simulink model "finalcode"  (R2020a)
settings: Solver=FixedStepDiscrete  StartTime=0.0  StopTime=1  FixedStep=0.0005  RelTol=1e-3  EnableMultiTasking=on
undefined symbols (not defined in the file): acc_calmax1, acc_calmax2, acc_calmin1, acc_calmin2, akemancanshu, angle_middle, bre, bre_calmax, bre_calmin, chasuniujvvvv_hou, chasuniujvvvv_qian, chasuuuu, ecucoder_acal, I_AN01_5K1, I_AN03_5V, I_AN04_5V, kd, kddd, ki, kiii, kp, kppp, leftmax, O_SW06_HS1A, P11111, P22222, PIDmodel, PPPP, rightmax, slip, slip_big, slip_little, slipmodel, T_add, T_del, tiaoshi, TTTTTyouren, vvvv, zhiling
libraries: ec5744lib x305, canmsglib x97, simulink x23
(part 5 of 11)

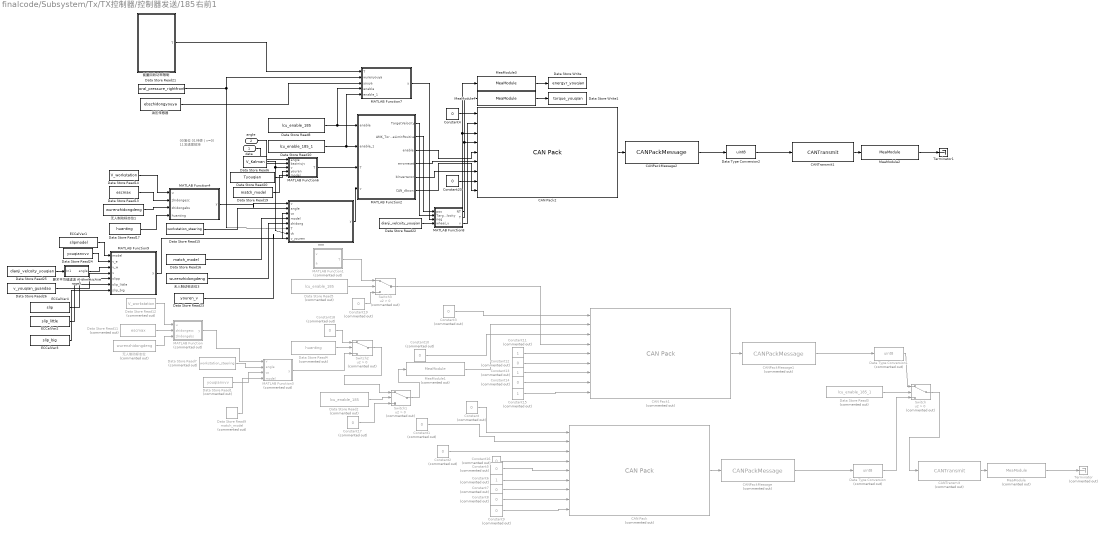
== system finalcode/Subsystem/Tx/TX控制器/控制器发送/185右前1 ==
  note: 00复位
      | 01待使（v=0)
      | 11发速度扭矩
  data : Inport
  angle : Inport  Port=2
  CAN Pack : canmsglib/CAN Pack  Commented=on  CANdbFile=D:\desktop\CANdbc\enable - youqian.dbc  MsgList=(none)  MsgName=first_enable  MsgIDType=Standard (11-bit identifier)  MsgIdentifier=389  MsgLength=8  Remote=off  ApplyMinMax=off  BusOutput=off  SignalInfo={'AMK_Reserve','12','4','LE','signed','Standard','0','1','0','0','15';'AMK_TargetVelocity','16','16','LE','signed','Standard','0','1','0','0','65535';'AMK_TorqueLimitNegativ','48','16','LE','signed','Standard','0','1','0','0','65535';'AMK_TorqueLimitPositiv','32','16','LE','signed','Standard','0','1','0','0','65535';'AMK_bEnable','10','1','LE','unsigned','Standard','0','1','0','0','1';'AMK_bErrorReset','11','1','LE','unsigned','Standard','0','1','0','0','1';'AMK_bInverterOn','8','1','LE','unsigned','Standard','0','1','0','0','1';'AMK_bReserve','0','8','LE','unsigned','Standard','0','1','0','0','255';'CAN_bdcon','9','1','LE','unsigned','Standard','0','1','0','0','1'}
      settings: SourceProductBaseCode=ME,XP,VN  DataFormat=CANdb specified signals
  CAN Pack1 : canmsglib/CAN Pack  Commented=on  CANdbFile=D:\desktop\CANdbc\enable - youqian.dbc  MsgList=(none)  MsgName=first_enable  MsgIDType=Standard (11-bit identifier)  MsgIdentifier=389  MsgLength=8  Remote=off  ApplyMinMax=off  BusOutput=off  SignalInfo={'AMK_Reserve','12','4','LE','signed','Standard','0','1','0','0','15';'AMK_TargetVelocity','16','16','LE','signed','Standard','0','1','0','0','65535';'AMK_TorqueLimitNegativ','48','16','LE','signed','Standard','0','1','0','0','65535';'AMK_TorqueLimitPositiv','32','16','LE','signed','Standard','0','1','0','0','65535';'AMK_bEnable','10','1','LE','unsigned','Standard','0','1','0','0','1';'AMK_bErrorReset','11','1','LE','unsigned','Standard','0','1','0','0','1';'AMK_bInverterOn','8','1','LE','unsigned','Standard','0','1','0','0','1';'AMK_bReserve','0','8','LE','unsigned','Standard','0','1','0','0','255';'CAN_bdcon','9','1','LE','unsigned','Standard','0','1','0','0','1'}
      settings: SourceProductBaseCode=ME,XP,VN  DataFormat=CANdb specified signals
  CAN Pack2 : canmsglib/CAN Pack  CANdbFile=C:\Users\86155\Desktop\HRT2024\qkx\can\enable_youqian.dbc  MsgList=first_enable  MsgName=first_enable  MsgIDType=Standard (11-bit identifier)  MsgIdentifier=389  MsgLength=8  Remote=off  ApplyMinMax=off  BusOutput=off  SignalInfo={'AMK_Reserve','12','4','LE','signed','Standard','0','1','0','-8','7';'AMK_TargetVelocity','16','16','LE','signed','Standard','0','1','0','-32768','32767';'AMK_TorqueLimitNegativ','48','16','LE','signed','Standard','0','1','0','-32768','32767';'AMK_TorqueLimitPositiv','32','16','LE','signed','Standard','0','1','0','-32768','32767';'AMK_bEnable','10','1','LE','unsigned','Standard','0','1','0','0','1';'AMK_bErrorReset','11','1','LE','unsigned','Standard','0','1','0','0','1';'AMK_bInverterOn','8','1','LE','unsigned','Standard','0','1','0','0','1';'AMK_bReserve','0','8','LE','unsigned','Standard','0','1','0','0','255';'CAN_bdcon','9','1','LE','unsigned','Standard','0','1','0','0','1'}
      settings: SourceProductBaseCode=ME,XP,VN  DataFormat=CANdb specified signals
  CANPackMessage : ec5744lib/RapidECU_U4B/04CANCommunication/CANPackMessage  Commented=on  datalength=8  sampletime=-1
      settings: SourceProductName=ECUCoder for MPC5744
  CANPackMessage1 : ec5744lib/RapidECU_U4B/04CANCommunication/CANPackMessage  Commented=on  datalength=8  sampletime=-1
      settings: SourceProductName=ECUCoder for MPC5744
  CANPackMessage2 : ec5744lib/RapidECU_U4B/04CANCommunication/CANPackMessage  datalength=8  sampletime=-1
      settings: SourceProductName=ECUCoder for MPC5744
  CANTransmit : ec5744lib/RapidECU_U4B/04CANCommunication/CANTransmit  Commented=on  canmodule=0  canbuffer=11  canmessageid=hex2dec('185')  canmessagetype=Standard(11-bit ID)  datalength=8  sampletime=-1
      settings: SourceProductName=ECUCoder for MPC5744
  CANTransmit1 : ec5744lib/RapidECU_U4B/04CANCommunication/CANTransmit  canmodule=0  canbuffer=11  canmessageid=hex2dec('185')  canmessagetype=Standard(11-bit ID)  datalength=8  sampletime=-1
      settings: SourceProductName=ECUCoder for MPC5744
  Constant{,1..3,5,7..10,12,14,16..17,19} (14 alike) : Constant  Commented=on  Value=0  SampleTime=-1
  Constant{6,11,13,15} (4 alike) : Constant  Commented=on  SampleTime=-1
  Constant18 : Constant  Commented=on  Value=0
  Constant20 : Constant  Value=0  SampleTime=-1
  Constant4 : Constant  Value=0  SampleTime=-1
  Data Store Read1 : DataStoreRead  Commented=on  DataStoreName=youqianvvv
  Data Store Read10 : DataStoreRead  DataStoreName=lcu_enable_185_1
  Data Store Read11 : DataStoreRead  Commented=on  DataStoreName=escmax
  Data Store Read12 : DataStoreRead  Commented=on  DataStoreName=V_workstation
  Data Store Read13 : DataStoreRead  DataStoreName=escmax
  Data Store Read14 : DataStoreRead  DataStoreName=V_workstation
  Data Store Read15 : DataStoreRead  DataStoreName=workstation_steering
  Data Store Read16 : DataStoreRead  DataStoreName=match_model
  Data Store Read17 : DataStoreRead  DataStoreName=huanting
  Data Store Read19 : DataStoreRead  DataStoreName=match_model
  Data Store Read2 : DataStoreRead  Commented=on  DataStoreName=lcu_enable_185
  Data Store Read20 : DataStoreRead  DataStoreName=Tyouqian
  Data Store Read21 : DataStoreRead  DataStoreName=oral_pressure_rightfront
  Data Store Read22 : DataStoreRead  DataStoreName=dianji_velcoity_youqian
  Data Store Read23 : DataStoreRead  DataStoreName=youren_v
  Data Store Read24 : DataStoreRead  DataStoreName=youqianvvv
  Data Store Read25 : DataStoreRead  DataStoreName=dianji_velcoity_youqian
  Data Store Read26 : DataStoreRead  DataStoreName=v_youqian_guandao
  Data Store Read3 : DataStoreRead  Commented=on  DataStoreName=lcu_enable_185_1
  Data Store Read4 : DataStoreRead  Commented=on  DataStoreName=huanting
  Data Store Read5 : DataStoreRead  Commented=on  DataStoreName=lcu_enable_185
  Data Store Read6 : DataStoreRead  DataStoreName=V_Kalman
  Data Store Read7 : DataStoreRead  Commented=on  DataStoreName=workstation_steering
  Data Store Read8 : DataStoreRead  DataStoreName=lcu_enable_185
  Data Store Read9 : DataStoreRead  Commented=on  DataStoreName=match_model
  Data Store Write : DataStoreWrite  DataStoreName=energyr_youqian
  Data Store Write1 : DataStoreWrite  DataStoreName=torque_youqian
  Data Type Conversion : DataTypeConversion  Commented=on  OutDataTypeStr=uint8
  Data Type Conversion1 : DataTypeConversion  Commented=on  OutDataTypeStr=uint8
  Data Type Conversion2 : DataTypeConversion  OutDataTypeStr=uint8
  ECCalVar1 : Constant  InitFcn=ecucoder_acal;  Value=slipmodel  OutDataTypeStr=Inherit: Inherit via back propagation  SampleTime=-1
  ECCalVar2 : Constant  InitFcn=ecucoder_acal;  Value=slip_little  OutDataTypeStr=Inherit: Inherit via back propagation  SampleTime=-1
  ECCalVar3 : Constant  InitFcn=ecucoder_acal;  Value=slip_big  OutDataTypeStr=Inherit: Inherit via back propagation  SampleTime=-1
  ECCalVar4 : Constant  InitFcn=ecucoder_acal;  Value=slip  OutDataTypeStr=Inherit: Inherit via back propagation  SampleTime=-1
  MATLAB Function : MATLAB Function  Commented=on  TreatAsAtomicUnit=on
  MATLAB Function1 : MATLAB Function  Commented=on  TreatAsAtomicUnit=on
  MATLAB Function2 : MATLAB Function  TreatAsAtomicUnit=on
  MATLAB Function3 : MATLAB Function  Commented=on  TreatAsAtomicUnit=on
  MATLAB Function4 : MATLAB Function  TreatAsAtomicUnit=on
  MATLAB Function6 : MATLAB Function  TreatAsAtomicUnit=on
  MATLAB Function7 : MATLAB Function  TreatAsAtomicUnit=on
  MATLAB Function8 : MATLAB Function  TreatAsAtomicUnit=on
  MATLAB Function9 : MATLAB Function  TreatAsAtomicUnit=on
  MeaModule : ec5744lib/RapidECU_U4B/07Calibration/MeaModule  Commented=on  signal=V185
      settings: SourceProductName=ECUCoder for MPC5744
  MeaModule1 : ec5744lib/RapidECU_U4B/07Calibration/MeaModule  Commented=on  signal=Vforth
      settings: SourceProductName=ECUCoder for MPC5744
  MeaModule2 : ec5744lib/RapidECU_U4B/07Calibration/MeaModule  signal=V185
      settings: SourceProductName=ECUCoder for MPC5744
  MeaModule3 : ec5744lib/RapidECU_U4B/07Calibration/MeaModule  signal=NT_youqian
      settings: SourceProductName=ECUCoder for MPC5744
  MeaModule4 : ec5744lib/RapidECU_U4B/07Calibration/MeaModule  signal=T_youqian
      settings: SourceProductName=ECUCoder for MPC5744
  Switch{,1..3} (4 alike) : Switch  Commented=on  Criteria=u2 > Threshold
  Terminator : Terminator  Commented=on
  Terminator1 : Terminator
  vvv : MATLAB Function  TreatAsAtomicUnit=on
  无人制动标志位 : DataStoreRead  Commented=on  DataStoreName=wurenzhidongdeng
  无人制动标志位1 : DataStoreRead  DataStoreName=wurenzhidongdeng
  无人制动标志位3 : DataStoreRead  DataStoreName=wurenzhidongdeng
  油压传感器 : DataStoreRead  DataStoreName=ebszhidongyouya
  算术平均值滤波 ArithmeticAverage5 : Subsystem
  能量回收功率限制 : Subsystem
  wires:
  Data Store Read10/1 -> MATLAB Function7/5(enable_1), MATLAB Function2/2(enable_1)
  Data Type Conversion2/1 -> CANTransmit1/1
  CAN Pack2/1 -> CANPackMessage2/1
  MeaModule2/1 -> Terminator1/1
  CANTransmit1/1 -> MeaModule2/1
  CANPackMessage2/1 -> Data Type Conversion2/1
  Data Store Read17/1 -> MATLAB Function4/4(huanting)
  vvv/1(y) -> MATLAB Function2/4(v)
  无人制动标志位1/1 -> MATLAB Function4/3(zhidongebs)
  Data Store Read14/1 -> MATLAB Function4/1(u)
  Data Store Read15/1 -> vvv/2(angle)
  Data Store Read13/1 -> MATLAB Function4/2(zhidongesc)
  Data Store Read16/1 -> vvv/4(model)
  MATLAB Function6/1(T) -> MATLAB Function2/3(T)
  Data Store Read8/1 -> MATLAB Function7/4(enable), MATLAB Function2/1("enable ")
  MATLAB Function2/4(errorreset) -> CAN Pack2/6
  Constant4/1 -> CAN Pack2/1
  MATLAB Function2/2(AMK_TorqueLimitPositive) -> MATLAB Function8/1(pos)
  MATLAB Function2/6(CAN_dbcon) -> CAN Pack2/9
  Constant20/1 -> CAN Pack2/8
  MATLAB Function2/5(blnverteron) -> CAN Pack2/7
  MATLAB Function2/3(enable) -> CAN Pack2/5
  Data Store Read12/1 -> MATLAB Function/1(u)
  Data Store Read11/1 -> MATLAB Function/2(zhidongesc)
  MATLAB Function/1(y) -> MATLAB Function3/1(v)
  无人制动标志位/1 -> MATLAB Function/3(zhidongebs)
  MATLAB Function1/1(T) -> Switch3/1
  Data Store Read9/1 -> MATLAB Function3/4(model)
  MATLAB Function3/1(y) -> Switch2/3
  Data Store Read1/1 -> MATLAB Function3/3(vz)
  Data Store Read7/1 -> MATLAB Function3/2(angle)
  Data Store Read5/1 -> Switch3/2
  Switch3/1 -> CAN Pack1/4
  Constant19/1 -> Switch3/3
  MeaModule1/1 -> CAN Pack1/2
  Switch2/1 -> Switch1/1
  Constant18/1 -> Switch2/1
  Data Store Read4/1 -> Switch2/2
  Data Store Read2/1 -> Switch1/2
  Constant17/1 -> Switch1/3
  Switch1/1 -> MeaModule1/1
  Data Store Read3/1 -> Switch/2
  Switch/1 -> CANTransmit/1
  Data Type Conversion/1 -> Switch/3
  Data Type Conversion1/1 -> Switch/1
  Constant15/1 -> CAN Pack1/9
  Constant14/1 -> CAN Pack1/8
  Constant10/1 -> CAN Pack1/3
  CAN Pack1/1 -> CANPackMessage1/1
  Constant13/1 -> CAN Pack1/7
  Constant12/1 -> CAN Pack1/6
  Constant11/1 -> CAN Pack1/5
  Constant3/1 -> CAN Pack1/1
  CANPackMessage1/1 -> Data Type Conversion1/1
  MeaModule/1 -> Terminator/1
  CANTransmit/1 -> MeaModule/1
  Constant6/1 -> CAN Pack/6
  Constant2/1 -> CAN Pack/3
  Constant16/1 -> CAN Pack/4
  Constant1/1 -> CAN Pack/2
  Constant7/1 -> CAN Pack/7
  CAN Pack/1 -> CANPackMessage/1
  Constant9/1 -> CAN Pack/9
  CANPackMessage/1 -> Data Type Conversion/1
  Constant/1 -> CAN Pack/1
  Constant5/1 -> CAN Pack/5
  Constant8/1 -> CAN Pack/8
  Data Store Read19/1 -> MATLAB Function6/5(model)
  Data Store Read20/1 -> MATLAB Function6/4(youren)
  Data Store Read6/1 -> vvv/7(vk), MATLAB Function6/3(v)
  MATLAB Function4/1(y) -> vvv/1(v)
  无人制动标志位3/1 -> vvv/5(zhidong)
  能量回收功率限制/1(T) -> MATLAB Function7/1(T)
  油压传感器/1 -> MATLAB Function7/3(youya)
  Data Store Read21/1 -> vvv/6(T), MATLAB Function7/2(wurenyouya)
  MATLAB Function7/1(y) -> MATLAB Function8/3(neg)
  Data Store Read23/1 -> vvv/8(v_youren)
  MATLAB Function2/1(TargetVelocity) -> MATLAB Function8/2(TargetVelocity)
  MATLAB Function8/3(v) -> CAN Pack2/2
  Data Store Read22/1 -> MATLAB Function8/4(wheel_v)
  MeaModule4/1 -> Data Store Write1/1
  MeaModule3/1 -> Data Store Write/1
  MATLAB Function8/2(T) -> MeaModule4/1, CAN Pack2/4
  MATLAB Function8/1(NT) -> MeaModule3/1, CAN Pack2/3
  Data Store Read26/1 -> MATLAB Function9/4(v)
  Data Store Read25/1 -> 算术平均值滤波 ArithmeticAverage5/1(In1)
  Data Store Read24/1 -> MATLAB Function9/2(v_e)
  算术平均值滤波 ArithmeticAverage5/1(angle) -> MATLAB Function9/3(v_w)
  MATLAB Function9/1(y) -> vvv/3(vz)
  data/1 -> MATLAB Function6/2(baziniujv)
  angle/1 -> MATLAB Function6/1(angle)
  ECCalVar1/1 -> MATLAB Function9/1(model)
  ECCalVar4/1 -> MATLAB Function9/5(slipp)
  ECCalVar2/1 -> MATLAB Function9/6(slip_little)
  ECCalVar3/1 -> MATLAB Function9/7(slip_big)

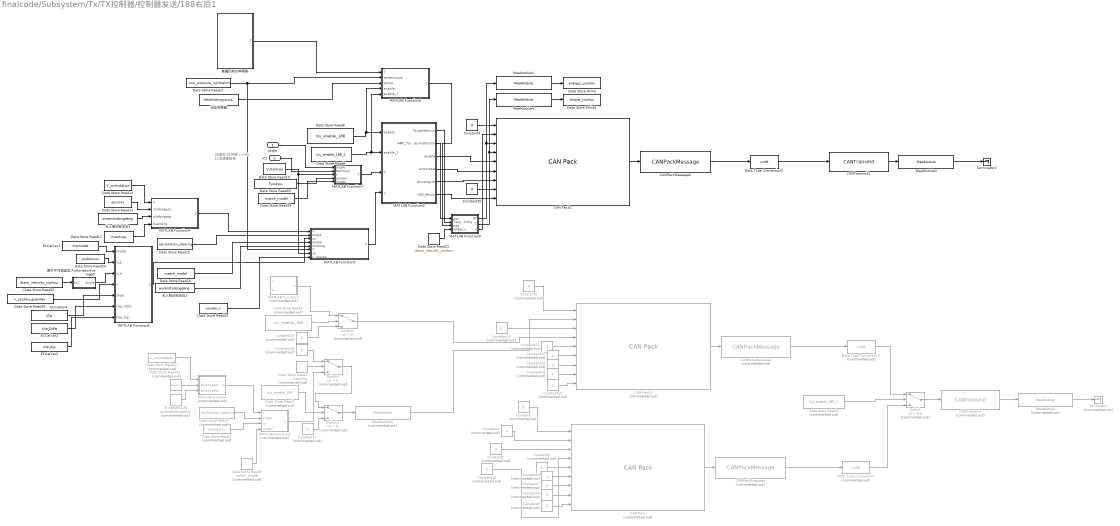
== system finalcode/Subsystem/Tx/TX控制器/控制器发送/188右后1 ==
  note: 00复位
      | 01待使（v=0)
      | 11发速度扭矩
  angle : Inport
  In1 : Inport  Port=2
  CAN Pack : canmsglib/CAN Pack  Commented=on  CANdbFile=D:\desktop\CANdbc\enable - zuohou - 副本.dbc  MsgList=(none)  MsgName=first_enable  MsgIDType=Standard (11-bit identifier)  MsgIdentifier=392  MsgLength=8  Remote=off  ApplyMinMax=off  BusOutput=off  SignalInfo={'AMK_Reserve','12','4','LE','signed','Standard','0','1','0','0','15';'AMK_TargetVelocity','16','16','LE','signed','Standard','0','1','0','0','65535';'AMK_TorqueLimitNegativ','48','16','LE','signed','Standard','0','1','0','0','65535';'AMK_TorqueLimitPositiv','32','16','LE','signed','Standard','0','1','0','0','65535';'AMK_bEnable','10','1','LE','unsigned','Standard','0','1','0','0','1';'AMK_bErrorReset','11','1','LE','unsigned','Standard','0','1','0','0','1';'AMK_bInverterOn','8','1','LE','unsigned','Standard','0','1','0','0','1';'AMK_bReserve','0','8','LE','unsigned','Standard','0','1','0','0','255';'CAN_bdcon','9','1','LE','unsigned','Standard','0','1','0','0','1'}
      settings: SourceProductBaseCode=ME,XP,VN  DataFormat=CANdb specified signals
  CAN Pack1 : canmsglib/CAN Pack  Commented=on  CANdbFile=D:\desktop\CANdbc\enable - zuohou - 副本.dbc  MsgList=(none)  MsgName=first_enable  MsgIDType=Standard (11-bit identifier)  MsgIdentifier=392  MsgLength=8  Remote=off  ApplyMinMax=off  BusOutput=off  SignalInfo={'AMK_Reserve','12','4','LE','signed','Standard','0','1','0','0','15';'AMK_TargetVelocity','16','16','LE','signed','Standard','0','1','0','0','65535';'AMK_TorqueLimitNegativ','48','16','LE','signed','Standard','0','1','0','0','65535';'AMK_TorqueLimitPositiv','32','16','LE','signed','Standard','0','1','0','0','65535';'AMK_bEnable','10','1','LE','unsigned','Standard','0','1','0','0','1';'AMK_bErrorReset','11','1','LE','unsigned','Standard','0','1','0','0','1';'AMK_bInverterOn','8','1','LE','unsigned','Standard','0','1','0','0','1';'AMK_bReserve','0','8','LE','unsigned','Standard','0','1','0','0','255';'CAN_bdcon','9','1','LE','unsigned','Standard','0','1','0','0','1'}
      settings: SourceProductBaseCode=ME,XP,VN  DataFormat=CANdb specified signals
  CAN Pack2 : canmsglib/CAN Pack  CANdbFile=C:\Users\86155\Desktop\HRT2024\qkx\can\enable_youhou.dbc  MsgList=first_enable  MsgName=first_enable  MsgIDType=Standard (11-bit identifier)  MsgIdentifier=392  MsgLength=8  Remote=off  ApplyMinMax=off  BusOutput=off  SignalInfo={'AMK_Reserve','12','4','LE','signed','Standard','0','1','0','-8','7';'AMK_TargetVelocity','16','16','LE','signed','Standard','0','1','0','-32768','32767';'AMK_TorqueLimitNegativ','48','16','LE','signed','Standard','0','1','0','-32768','32767';'AMK_TorqueLimitPositiv','32','16','LE','signed','Standard','0','1','0','-32768','32767';'AMK_bEnable','10','1','LE','unsigned','Standard','0','1','0','0','1';'AMK_bErrorReset','11','1','LE','unsigned','Standard','0','1','0','0','1';'AMK_bInverterOn','8','1','LE','unsigned','Standard','0','1','0','0','1';'AMK_bReserve','0','8','LE','unsigned','Standard','0','1','0','0','255';'CAN_bdcon','9','1','LE','unsigned','Standard','0','1','0','0','1'}
      settings: SourceProductBaseCode=ME,XP,VN  DataFormat=CANdb specified signals
  CANPackMessage : ec5744lib/RapidECU_U4B/04CANCommunication/CANPackMessage  Commented=on  datalength=8  sampletime=-1
      settings: SourceProductName=ECUCoder for MPC5744
  CANPackMessage1 : ec5744lib/RapidECU_U4B/04CANCommunication/CANPackMessage  Commented=on  datalength=8  sampletime=-1
      settings: SourceProductName=ECUCoder for MPC5744
  CANPackMessage2 : ec5744lib/RapidECU_U4B/04CANCommunication/CANPackMessage  datalength=8  sampletime=-1
      settings: SourceProductName=ECUCoder for MPC5744
  CANTransmit : ec5744lib/RapidECU_U4B/04CANCommunication/CANTransmit  Commented=on  canmodule=0  canbuffer=9  canmessageid=hex2dec('188')  canmessagetype=Standard(11-bit ID)  datalength=8  sampletime=-1
      settings: SourceProductName=ECUCoder for MPC5744
  CANTransmit1 : ec5744lib/RapidECU_U4B/04CANCommunication/CANTransmit  canmodule=0  canbuffer=9  canmessageid=hex2dec('188')  canmessagetype=Standard(11-bit ID)  datalength=8  sampletime=-1
      settings: SourceProductName=ECUCoder for MPC5744
  Constant{,1..3,5,7..10,12,14,17,19} (13 alike) : Constant  Commented=on  Value=0  SampleTime=-1
  Constant{6,11,13,15} (4 alike) : Constant  Commented=on  SampleTime=-1
  Constant16 : Constant  Commented=on  Value=0
  Constant18 : Constant  Commented=on  Value=0
  Constant20 : Constant  Value=0  SampleTime=-1
  Constant4 : Constant  Value=0  SampleTime=-1
  Data Store Read1 : DataStoreRead  Commented=on  DataStoreName=lcu_enable_188
  Data Store Read10 : DataStoreRead  DataStoreName=V_Kalman
  Data Store Read11 : DataStoreRead  Commented=on  DataStoreName=escmax
  Data Store Read12 : DataStoreRead  Commented=on  DataStoreName=V_workstation
  Data Store Read13 : DataStoreRead  DataStoreName=escmax
  Data Store Read14 : DataStoreRead  DataStoreName=V_workstation
  Data Store Read15 : DataStoreRead  DataStoreName=workstation_steering
  Data Store Read16 : DataStoreRead  DataStoreName=match_model
  Data Store Read17 : DataStoreRead  DataStoreName=huanting
  Data Store Read19 : DataStoreRead  DataStoreName=match_model
  Data Store Read2 : DataStoreRead  Commented=on  DataStoreName=youhouvvv
  Data Store Read20 : DataStoreRead  DataStoreName=Tyouhou
  Data Store Read21 : DataStoreRead  DataStoreName=oral_pressure_rightbehind
  Data Store Read22 : DataStoreRead  DataStoreName=dianji_velcoity_youhou
  Data Store Read23 : DataStoreRead  DataStoreName=youren_v
  Data Store Read24 : DataStoreRead  DataStoreName=youhouvvv
  Data Store Read25 : DataStoreRead  DataStoreName=dianji_velcoity_zuohou
  Data Store Read26 : DataStoreRead  DataStoreName=v_youhou_guandao
  Data Store Read3 : DataStoreRead  Commented=on  DataStoreName=lcu_enable_188_1
  Data Store Read4 : DataStoreRead  Commented=on  DataStoreName=huanting
  Data Store Read5 : DataStoreRead  Commented=on  DataStoreName=lcu_enable_188
  Data Store Read6 : DataStoreRead  DataStoreName=lcu_enable_188_1
  Data Store Read7 : DataStoreRead  Commented=on  DataStoreName=workstation_steering
  Data Store Read8 : DataStoreRead  DataStoreName=lcu_enable_188
  Data Store Read9 : DataStoreRead  Commented=on  DataStoreName=match_model
  Data Store Write : DataStoreWrite  DataStoreName=energyr_youhou
  Data Store Write1 : DataStoreWrite  DataStoreName=torque_youhou
  Data Type Conversion : DataTypeConversion  Commented=on  OutDataTypeStr=uint8
  Data Type Conversion1 : DataTypeConversion  Commented=on  OutDataTypeStr=uint8
  Data Type Conversion2 : DataTypeConversion  OutDataTypeStr=uint8
  ECCalVar1 : Constant  InitFcn=ecucoder_acal;  Value=slipmodel  OutDataTypeStr=Inherit: Inherit via back propagation  SampleTime=-1
  ECCalVar2 : Constant  InitFcn=ecucoder_acal;  Value=slip_little  OutDataTypeStr=Inherit: Inherit via back propagation  SampleTime=-1
  ECCalVar3 : Constant  InitFcn=ecucoder_acal;  Value=slip_big  OutDataTypeStr=Inherit: Inherit via back propagation  SampleTime=-1
  ECCalVar4 : Constant  InitFcn=ecucoder_acal;  Value=slip  OutDataTypeStr=Inherit: Inherit via back propagation  SampleTime=-1
  MATLAB Function : MATLAB Function  Commented=on  TreatAsAtomicUnit=on
  MATLAB Function1 : MATLAB Function  Commented=on  TreatAsAtomicUnit=on
  MATLAB Function2 : MATLAB Function  TreatAsAtomicUnit=on
  MATLAB Function3 : MATLAB Function  Commented=on  TreatAsAtomicUnit=on
  MATLAB Function4 : MATLAB Function  TreatAsAtomicUnit=on
  MATLAB Function5 : MATLAB Function  TreatAsAtomicUnit=on
  MATLAB Function6 : MATLAB Function  TreatAsAtomicUnit=on
  MATLAB Function7 : MATLAB Function  TreatAsAtomicUnit=on
  MATLAB Function8 : MATLAB Function  TreatAsAtomicUnit=on
  MATLAB Function9 : MATLAB Function  TreatAsAtomicUnit=on
  MeaModule : ec5744lib/RapidECU_U4B/07Calibration/MeaModule  Commented=on  signal=V188
      settings: SourceProductName=ECUCoder for MPC5744
  MeaModule1 : ec5744lib/RapidECU_U4B/07Calibration/MeaModule  Commented=on  signal=Vsecond
      settings: SourceProductName=ECUCoder for MPC5744
  MeaModule2 : ec5744lib/RapidECU_U4B/07Calibration/MeaModule  signal=NT_youhou
      settings: SourceProductName=ECUCoder for MPC5744
  MeaModule3 : ec5744lib/RapidECU_U4B/07Calibration/MeaModule  signal=V188
      settings: SourceProductName=ECUCoder for MPC5744
  MeaModule4 : ec5744lib/RapidECU_U4B/07Calibration/MeaModule  signal=T_youhou
      settings: SourceProductName=ECUCoder for MPC5744
  Switch : Switch  Commented=on  Criteria=u2 > Threshold  Threshold=0.9
  Switch1 : Switch  Commented=on  Criteria=u2 > Threshold
  Switch2 : Switch  Commented=on  Criteria=u2 > Threshold
  Switch3 : Switch  Commented=on  Criteria=u2 > Threshold
  Terminator : Terminator  Commented=on
  Terminator1 : Terminator
  无人制动标志位 : DataStoreRead  Commented=on  DataStoreName=wurenzhidongdeng
  无人制动标志位1 : DataStoreRead  DataStoreName=wurenzhidongdeng
  无人制动标志位3 : DataStoreRead  DataStoreName=wurenzhidongdeng
  油压传感器 : DataStoreRead  DataStoreName=ebszhidongyouya
  算术平均值滤波 ArithmeticAverage5 : Subsystem
  能量回收功率限制 : Subsystem
  wires:
  CANPackMessage2/1 -> Data Type Conversion2/1
  CAN Pack2/1 -> CANPackMessage2/1
  CANTransmit1/1 -> MeaModule3/1
  Data Store Read16/1 -> MATLAB Function5/4(model)
  Constant20/1 -> CAN Pack2/8
  Data Type Conversion2/1 -> CANTransmit1/1
  MATLAB Function7/1(T) -> MATLAB Function2/3(T)
  MeaModule3/1 -> Terminator1/1
  MATLAB Function2/5(blnverteron) -> CAN Pack2/7
  MATLAB Function2/4(errorreset) -> CAN Pack2/6
  MATLAB Function2/3(enable) -> CAN Pack2/5
  MATLAB Function2/6(CAN_dbcon) -> CAN Pack2/9
  MATLAB Function2/2(AMK_TorqueLimitPositive) -> MATLAB Function9/1(pos)
  Data Store Read6/1 -> MATLAB Function6/5(enable_1), MATLAB Function2/2(enable_1)
  Constant4/1 -> CAN Pack2/1
  Data Store Read8/1 -> MATLAB Function6/4(enable), MATLAB Function2/1("enable ")
  MATLAB Function5/1(y) -> MATLAB Function2/4(v)
  Data Store Read17/1 -> MATLAB Function4/4(huanting)
  Data Store Read13/1 -> MATLAB Function4/2(zhidongesc)
  MATLAB Function4/1(y) -> MATLAB Function5/1(v)
  无人制动标志位1/1 -> MATLAB Function4/3(zhidongebs)
  Data Store Read15/1 -> MATLAB Function5/2(angle)
  Data Store Read14/1 -> MATLAB Function4/1(u)
  Data Store Read2/1 -> MATLAB Function3/3(vz)
  Data Store Read12/1 -> MATLAB Function/1(u)
  Data Store Read11/1 -> MATLAB Function/2(zhidongesc)
  MATLAB Function/1(y) -> MATLAB Function3/1(v)
  无人制动标志位/1 -> MATLAB Function/3(zhidongebs)
  MATLAB Function1/1(T) -> Switch3/1
  Data Store Read9/1 -> MATLAB Function3/4(model)
  MATLAB Function3/1(y) -> Switch2/3
  Data Store Read7/1 -> MATLAB Function3/2(angle)
  Data Store Read5/1 -> Switch3/2
  Constant19/1 -> Switch3/3
  Switch3/1 -> CAN Pack1/4
  MeaModule1/1 -> CAN Pack1/2
  Switch2/1 -> Switch1/1
  Constant18/1 -> Switch2/1
  Data Store Read4/1 -> Switch2/2
  Switch1/1 -> MeaModule1/1
  Data Store Read1/1 -> Switch1/2
  Constant17/1 -> Switch1/3
  Switch/1 -> CANTransmit/1
  Data Type Conversion/1 -> Switch/3
  Data Store Read3/1 -> Switch/2
  Constant13/1 -> CAN Pack1/7
  Constant15/1 -> CAN Pack1/9
  CAN Pack1/1 -> CANPackMessage1/1
  Constant11/1 -> CAN Pack1/5
  Constant3/1 -> CAN Pack1/1
  Constant14/1 -> CAN Pack1/8
  CANPackMessage1/1 -> Data Type Conversion1/1
  Constant10/1 -> CAN Pack1/3
  Constant12/1 -> CAN Pack1/6
  Data Type Conversion1/1 -> Switch/1
  MeaModule/1 -> Terminator/1
  CANTransmit/1 -> MeaModule/1
  Constant6/1 -> CAN Pack/6
  Constant2/1 -> CAN Pack/3
  Constant16/1 -> CAN Pack/4
  Constant1/1 -> CAN Pack/2
  Constant7/1 -> CAN Pack/7
  CAN Pack/1 -> CANPackMessage/1
  Constant9/1 -> CAN Pack/9
  CANPackMessage/1 -> Data Type Conversion/1
  Constant/1 -> CAN Pack/1
  Constant5/1 -> CAN Pack/5
  Constant8/1 -> CAN Pack/8
  Data Store Read19/1 -> MATLAB Function7/5(model)
  Data Store Read20/1 -> MATLAB Function7/4(youren)
  Data Store Read10/1 -> MATLAB Function7/3(v), MATLAB Function5/7(vk)
  无人制动标志位3/1 -> MATLAB Function5/5(zhidong)
  能量回收功率限制/1(T) -> MATLAB Function6/1(T)
  油压传感器/1 -> MATLAB Function6/3(youya)
  Data Store Read21/1 -> MATLAB Function5/6(T), MATLAB Function6/2(wurenyouya)
  MATLAB Function6/1(y) -> MATLAB Function9/3(neg)
  Data Store Read23/1 -> MATLAB Function5/8(v_youren)
  MATLAB Function2/1(TargetVelocity) -> MATLAB Function9/2(TargetVelocity)
  MATLAB Function9/3(v) -> CAN Pack2/2
  Data Store Read22/1 -> MATLAB Function9/4(wheel_v)
  MeaModule2/1 -> Data Store Write/1
  MeaModule4/1 -> Data Store Write1/1
  MATLAB Function9/2(T) -> MeaModule4/1, CAN Pack2/4
  MATLAB Function9/1(NT) -> MeaModule2/1, CAN Pack2/3
  Data Store Read26/1 -> MATLAB Function8/4(v)
  Data Store Read25/1 -> 算术平均值滤波 ArithmeticAverage5/1(In1)
  Data Store Read24/1 -> MATLAB Function8/2(v_e)
  算术平均值滤波 ArithmeticAverage5/1(angle) -> MATLAB Function8/3(v_w)
  MATLAB Function8/1(y) -> MATLAB Function5/3(vz)
  In1/1 -> MATLAB Function7/2(baziniujv)
  angle/1 -> MATLAB Function7/1(angle)
  ECCalVar1/1 -> MATLAB Function8/1(model)
  ECCalVar4/1 -> MATLAB Function8/5(slipp)
  ECCalVar2/1 -> MATLAB Function8/6(slip_little)
  ECCalVar3/1 -> MATLAB Function8/7(slip_big)

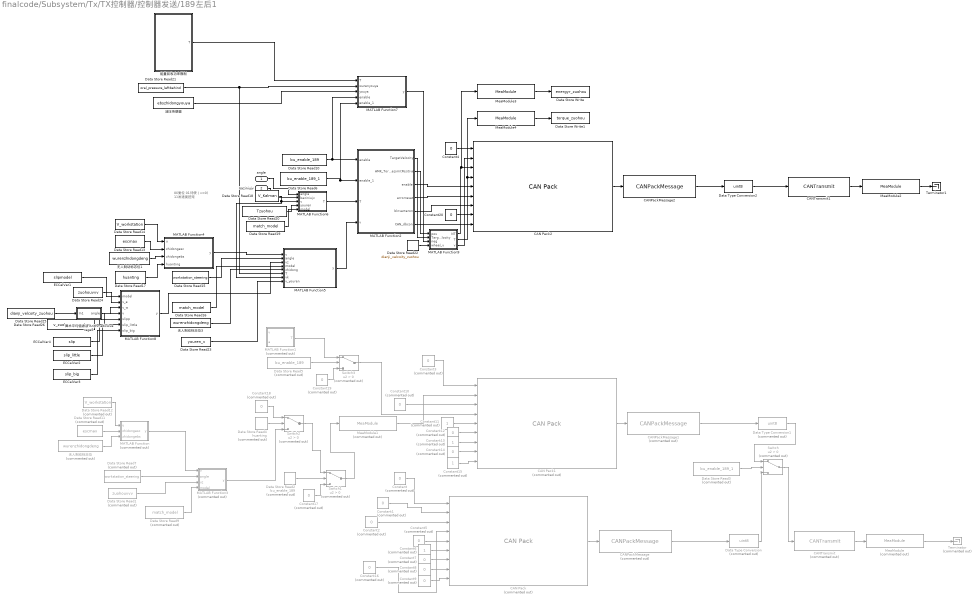
== system finalcode/Subsystem/Tx/TX控制器/控制器发送/189左后1 ==
  note: 00复位
      | 01待使（v=0)
      | 11发速度扭矩
  angle : Inport
  baziniujv : Inport  Port=2
  CAN Pack : canmsglib/CAN Pack  Commented=on  CANdbFile=D:\desktop\CANdbc\enable - youhou -.dbc  MsgList=(none)  MsgName=first_enable  MsgIDType=Standard (11-bit identifier)  MsgIdentifier=393  MsgLength=8  Remote=off  ApplyMinMax=off  BusOutput=off  SignalInfo={'AMK_Reserve','12','4','LE','signed','Standard','0','1','0','0','15';'AMK_TargetVelocity','16','16','LE','signed','Standard','0','1','0','0','65535';'AMK_TorqueLimitNegativ','48','16','LE','signed','Standard','0','1','0','0','65535';'AMK_TorqueLimitPositiv','32','16','LE','signed','Standard','0','1','0','0','65535';'AMK_bEnable','10','1','LE','unsigned','Standard','0','1','0','0','1';'AMK_bErrorReset','11','1','LE','unsigned','Standard','0','1','0','0','1';'AMK_bInverterOn','8','1','LE','unsigned','Standard','0','1','0','0','1';'AMK_bReserve','0','8','LE','unsigned','Standard','0','1','0','0','255';'CAN_bdcon','9','1','LE','unsigned','Standard','0','1','0','0','1'}
      settings: SourceProductBaseCode=ME,XP,VN  DataFormat=CANdb specified signals
  CAN Pack1 : canmsglib/CAN Pack  Commented=on  CANdbFile=D:\desktop\CANdbc\enable - youhou -.dbc  MsgList=(none)  MsgName=first_enable  MsgIDType=Standard (11-bit identifier)  MsgIdentifier=393  MsgLength=8  Remote=off  ApplyMinMax=off  BusOutput=off  SignalInfo={'AMK_Reserve','12','4','LE','signed','Standard','0','1','0','0','15';'AMK_TargetVelocity','16','16','LE','signed','Standard','0','1','0','0','65535';'AMK_TorqueLimitNegativ','48','16','LE','signed','Standard','0','1','0','0','65535';'AMK_TorqueLimitPositiv','32','16','LE','signed','Standard','0','1','0','0','65535';'AMK_bEnable','10','1','LE','unsigned','Standard','0','1','0','0','1';'AMK_bErrorReset','11','1','LE','unsigned','Standard','0','1','0','0','1';'AMK_bInverterOn','8','1','LE','unsigned','Standard','0','1','0','0','1';'AMK_bReserve','0','8','LE','unsigned','Standard','0','1','0','0','255';'CAN_bdcon','9','1','LE','unsigned','Standard','0','1','0','0','1'}
      settings: SourceProductBaseCode=ME,XP,VN  DataFormat=CANdb specified signals
  CAN Pack2 : canmsglib/CAN Pack  CANdbFile=C:\Users\86155\Desktop\HRT2024\qkx\can\enabe_zuohou.dbc  MsgList=first_enable  MsgName=first_enable  MsgIDType=Standard (11-bit identifier)  MsgIdentifier=393  MsgLength=8  Remote=off  ApplyMinMax=off  BusOutput=off  SignalInfo={'AMK_Reserve','12','4','LE','signed','Standard','0','1','0','-8','7';'AMK_TargetVelocity','16','16','LE','signed','Standard','0','1','0','-32768','32767';'AMK_TorqueLimitNegativ','48','16','LE','signed','Standard','0','1','0','-32768','32767';'AMK_TorqueLimitPositiv','32','16','LE','signed','Standard','0','1','0','-32768','32767';'AMK_bEnable','10','1','LE','unsigned','Standard','0','1','0','0','1';'AMK_bErrorReset','11','1','LE','unsigned','Standard','0','1','0','0','1';'AMK_bInverterOn','8','1','LE','unsigned','Standard','0','1','0','0','1';'AMK_bReserve','0','8','LE','unsigned','Standard','0','1','0','0','255';'CAN_bdcon','9','1','LE','unsigned','Standard','0','1','0','0','1'}
      settings: SourceProductBaseCode=ME,XP,VN  DataFormat=CANdb specified signals
  CANPackMessage : ec5744lib/RapidECU_U4B/04CANCommunication/CANPackMessage  Commented=on  datalength=8  sampletime=-1
      settings: SourceProductName=ECUCoder for MPC5744
  CANPackMessage1 : ec5744lib/RapidECU_U4B/04CANCommunication/CANPackMessage  Commented=on  datalength=8  sampletime=-1
      settings: SourceProductName=ECUCoder for MPC5744
  CANPackMessage2 : ec5744lib/RapidECU_U4B/04CANCommunication/CANPackMessage  datalength=8  sampletime=-1
      settings: SourceProductName=ECUCoder for MPC5744
  CANTransmit : ec5744lib/RapidECU_U4B/04CANCommunication/CANTransmit  Commented=on  canmodule=0  canbuffer=10  canmessageid=hex2dec('189')  canmessagetype=Standard(11-bit ID)  datalength=8  sampletime=-1
      settings: SourceProductName=ECUCoder for MPC5744
  CANTransmit1 : ec5744lib/RapidECU_U4B/04CANCommunication/CANTransmit  canmodule=0  canbuffer=10  canmessageid=hex2dec('189')  canmessagetype=Standard(11-bit ID)  datalength=8  sampletime=-1
      settings: SourceProductName=ECUCoder for MPC5744
  Constant{,1..3,5,7..10,12,14,16..17,19} (14 alike) : Constant  Commented=on  Value=0  SampleTime=-1
  Constant{6,11,13,15} (4 alike) : Constant  Commented=on  SampleTime=-1
  Constant18 : Constant  Commented=on  Value=0
  Constant20 : Constant  Value=0  SampleTime=-1
  Constant4 : Constant  Value=0  SampleTime=-1
  Data Store Read1 : DataStoreRead  Commented=on  DataStoreName=zuohouvvv
  Data Store Read10 : DataStoreRead  DataStoreName=lcu_enable_189
  Data Store Read11 : DataStoreRead  Commented=on  DataStoreName=escmax
  Data Store Read12 : DataStoreRead  Commented=on  DataStoreName=V_workstation
  Data Store Read13 : DataStoreRead  DataStoreName=escmax
  Data Store Read14 : DataStoreRead  DataStoreName=V_workstation
  Data Store Read15 : DataStoreRead  DataStoreName=workstation_steering
  Data Store Read16 : DataStoreRead  DataStoreName=match_model
  Data Store Read17 : DataStoreRead  DataStoreName=huanting
  Data Store Read18 : DataStoreRead  DataStoreName=V_Kalman
  Data Store Read19 : DataStoreRead  DataStoreName=match_model
  Data Store Read2 : DataStoreRead  Commented=on  DataStoreName=lcu_enable_189
  Data Store Read20 : DataStoreRead  DataStoreName=Tzuohou
  Data Store Read21 : DataStoreRead  DataStoreName=oral_pressure_leftbehind
  Data Store Read22 : DataStoreRead  DataStoreName=dianji_velcoity_zuohou
  Data Store Read23 : DataStoreRead  DataStoreName=youren_v
  Data Store Read24 : DataStoreRead  DataStoreName=zuohouvvv
  Data Store Read25 : DataStoreRead  DataStoreName=dianji_velcoity_zuohou
  Data Store Read26 : DataStoreRead  DataStoreName=v_zuohou_guandao
  Data Store Read3 : DataStoreRead  Commented=on  DataStoreName=lcu_enable_189_1
  Data Store Read4 : DataStoreRead  Commented=on  DataStoreName=huanting
  Data Store Read5 : DataStoreRead  Commented=on  DataStoreName=lcu_enable_189
  Data Store Read6 : DataStoreRead  DataStoreName=lcu_enable_189_1
  Data Store Read7 : DataStoreRead  Commented=on  DataStoreName=workstation_steering
  Data Store Read9 : DataStoreRead  Commented=on  DataStoreName=match_model
  Data Store Write : DataStoreWrite  DataStoreName=energyr_zuohou
  Data Store Write1 : DataStoreWrite  DataStoreName=torque_zuohou
  Data Type Conversion : DataTypeConversion  Commented=on  OutDataTypeStr=uint8
  Data Type Conversion1 : DataTypeConversion  Commented=on  OutDataTypeStr=uint8
  Data Type Conversion2 : DataTypeConversion  OutDataTypeStr=uint8
  ECCalVar1 : Constant  InitFcn=ecucoder_acal;  Value=slipmodel  OutDataTypeStr=Inherit: Inherit via back propagation  SampleTime=-1
  ECCalVar2 : Constant  InitFcn=ecucoder_acal;  Value=slip_little  OutDataTypeStr=Inherit: Inherit via back propagation  SampleTime=-1
  ECCalVar3 : Constant  InitFcn=ecucoder_acal;  Value=slip_big  OutDataTypeStr=Inherit: Inherit via back propagation  SampleTime=-1
  ECCalVar4 : Constant  InitFcn=ecucoder_acal;  Value=slip  OutDataTypeStr=Inherit: Inherit via back propagation  SampleTime=-1
  MATLAB Function : MATLAB Function  Commented=on  TreatAsAtomicUnit=on
  MATLAB Function1 : MATLAB Function  Commented=on  TreatAsAtomicUnit=on
  MATLAB Function2 : MATLAB Function  TreatAsAtomicUnit=on
  MATLAB Function3 : MATLAB Function  Commented=on  TreatAsAtomicUnit=on
  MATLAB Function4 : MATLAB Function  TreatAsAtomicUnit=on
  MATLAB Function5 : MATLAB Function  TreatAsAtomicUnit=on
  MATLAB Function6 : MATLAB Function  TreatAsAtomicUnit=on
  MATLAB Function7 : MATLAB Function  TreatAsAtomicUnit=on
  MATLAB Function8 : MATLAB Function  TreatAsAtomicUnit=on
  MATLAB Function9 : MATLAB Function  TreatAsAtomicUnit=on
  MeaModule : ec5744lib/RapidECU_U4B/07Calibration/MeaModule  Commented=on  signal=V189
      settings: SourceProductName=ECUCoder for MPC5744
  MeaModule1 : ec5744lib/RapidECU_U4B/07Calibration/MeaModule  Commented=on  signal=Vthird
      settings: SourceProductName=ECUCoder for MPC5744
  MeaModule2 : ec5744lib/RapidECU_U4B/07Calibration/MeaModule  signal=V189
      settings: SourceProductName=ECUCoder for MPC5744
  MeaModule3 : ec5744lib/RapidECU_U4B/07Calibration/MeaModule  signal=NT_zuohou
      settings: SourceProductName=ECUCoder for MPC5744
  MeaModule4 : ec5744lib/RapidECU_U4B/07Calibration/MeaModule  signal=T_zuohou
      settings: SourceProductName=ECUCoder for MPC5744
  Switch{,1..3} (4 alike) : Switch  Commented=on  Criteria=u2 > Threshold
  Terminator : Terminator  Commented=on
  Terminator1 : Terminator
  无人制动标志位 : DataStoreRead  Commented=on  DataStoreName=wurenzhidongdeng
  无人制动标志位1 : DataStoreRead  DataStoreName=wurenzhidongdeng
  无人制动标志位3 : DataStoreRead  DataStoreName=wurenzhidongdeng
  油压传感器 : DataStoreRead  DataStoreName=ebszhidongyouya
  算术平均值滤波 ArithmeticAverage5 : Subsystem
  能量回收功率限制 : Subsystem
  wires:
  MeaModule2/1 -> Terminator1/1
  Data Type Conversion2/1 -> CANTransmit1/1
  CANPackMessage2/1 -> Data Type Conversion2/1
  CAN Pack2/1 -> CANPackMessage2/1
  CANTransmit1/1 -> MeaModule2/1
  MATLAB Function2/5(blnverteron) -> CAN Pack2/7
  Data Store Read10/1 -> MATLAB Function7/4(enable), MATLAB Function2/1("enable ")
  Data Store Read17/1 -> MATLAB Function4/4(huanting)
  Constant4/1 -> CAN Pack2/1
  Data Store Read16/1 -> MATLAB Function5/4(model)
  Data Store Read6/1 -> MATLAB Function7/5(enable_1), MATLAB Function2/2(enable_1)
  MATLAB Function2/4(errorreset) -> CAN Pack2/6
  MATLAB Function2/2(AMK_TorqueLimitPositive) -> MATLAB Function9/1(pos)
  MATLAB Function2/6(CAN_dbcon) -> CAN Pack2/9
  MATLAB Function2/3(enable) -> CAN Pack2/5
  MATLAB Function2/1(TargetVelocity) -> MATLAB Function9/2(TargetVelocity)
  Constant20/1 -> CAN Pack2/8
  MATLAB Function4/1(y) -> MATLAB Function5/1(v)
  Data Store Read14/1 -> MATLAB Function4/1(u)
  Data Store Read15/1 -> MATLAB Function5/2(angle)
  无人制动标志位1/1 -> MATLAB Function4/3(zhidongebs)
  Data Store Read13/1 -> MATLAB Function4/2(zhidongesc)
  Data Store Read1/1 -> MATLAB Function3/3(vz)
  Data Store Read12/1 -> MATLAB Function/1(u)
  Data Store Read11/1 -> MATLAB Function/2(zhidongesc)
  无人制动标志位/1 -> MATLAB Function/3(zhidongebs)
  MATLAB Function1/1(T) -> Switch3/1
  Data Store Read9/1 -> MATLAB Function3/4(model)
  MATLAB Function/1(y) -> MATLAB Function3/1(v)
  MATLAB Function3/1(y) -> Switch2/3
  Data Store Read7/1 -> MATLAB Function3/2(angle)
  Data Store Read5/1 -> Switch3/2
  Switch3/1 -> CAN Pack1/4
  Constant19/1 -> Switch3/3
  MeaModule1/1 -> CAN Pack1/2
  Switch2/1 -> Switch1/1
  Constant18/1 -> Switch2/1
  Data Store Read4/1 -> Switch2/2
  Switch1/1 -> MeaModule1/1
  Data Store Read2/1 -> Switch1/2
  Constant17/1 -> Switch1/3
  Data Store Read3/1 -> Switch/2
  Switch/1 -> CANTransmit/1
  Data Type Conversion/1 -> Switch/3
  Data Type Conversion1/1 -> Switch/1
  Constant3/1 -> CAN Pack1/1
  Constant15/1 -> CAN Pack1/9
  CAN Pack1/1 -> CANPackMessage1/1
  CANPackMessage1/1 -> Data Type Conversion1/1
  Constant13/1 -> CAN Pack1/7
  Constant11/1 -> CAN Pack1/5
  Constant14/1 -> CAN Pack1/8
  Constant10/1 -> CAN Pack1/3
  Constant12/1 -> CAN Pack1/6
  MeaModule/1 -> Terminator/1
  CANTransmit/1 -> MeaModule/1
  Constant6/1 -> CAN Pack/6
  Constant2/1 -> CAN Pack/3
  Constant16/1 -> CAN Pack/4
  Constant1/1 -> CAN Pack/2
  Constant7/1 -> CAN Pack/7
  CAN Pack/1 -> CANPackMessage/1
  Constant9/1 -> CAN Pack/9
  CANPackMessage/1 -> Data Type Conversion/1
  Constant/1 -> CAN Pack/1
  Constant5/1 -> CAN Pack/5
  Constant8/1 -> CAN Pack/8
  Data Store Read19/1 -> MATLAB Function6/5(model)
  Data Store Read20/1 -> MATLAB Function6/4(youren)
  Data Store Read18/1 -> MATLAB Function5/7(vk), MATLAB Function6/3(v)
  MATLAB Function6/1(T) -> MATLAB Function2/3(T)
  MATLAB Function5/1(y) -> MATLAB Function2/4(v)
  无人制动标志位3/1 -> MATLAB Function5/5(zhidong)
  能量回收功率限制/1(T) -> MATLAB Function7/1(T)
  油压传感器/1 -> MATLAB Function7/3(youya)
  Data Store Read21/1 -> MATLAB Function5/6(T), MATLAB Function7/2(wurenyouya)
  MATLAB Function7/1(y) -> MATLAB Function9/3(neg)
  Data Store Read23/1 -> MATLAB Function5/8(v_youren)
  MATLAB Function9/3(v) -> CAN Pack2/2
  Data Store Read22/1 -> MATLAB Function9/4(wheel_v)
  MeaModule4/1 -> Data Store Write1/1
  MeaModule3/1 -> Data Store Write/1
  MATLAB Function9/2(T) -> MeaModule4/1, CAN Pack2/4
  MATLAB Function9/1(NT) -> MeaModule3/1, CAN Pack2/3
  Data Store Read26/1 -> MATLAB Function8/4(v)
  Data Store Read25/1 -> 算术平均值滤波 ArithmeticAverage5/1(In1)
  Data Store Read24/1 -> MATLAB Function8/2(v_e)
  算术平均值滤波 ArithmeticAverage5/1(angle) -> MATLAB Function8/3(v_w)
  MATLAB Function8/1(y) -> MATLAB Function5/3(vz)
  angle/1 -> MATLAB Function6/1(angle)
  baziniujv/1 -> MATLAB Function6/2(baziniujv)
  ECCalVar1/1 -> MATLAB Function8/1(model)
  ECCalVar4/1 -> MATLAB Function8/5(slipp)
  ECCalVar2/1 -> MATLAB Function8/6(slip_little)
  ECCalVar3/1 -> MATLAB Function8/7(slip_big)

== system finalcode/Subsystem/Tx/TX控制器/控制器发送/算术平均值滤波 ArithmeticAverage ==
  In1 : Inport
  Constant : Constant  Value=10
  Divide : Product  Inputs=*/
  Sum of Elements : Sum  Inputs=+
  Tapped Delay : simulink/Discrete/Tapped Delay  vinit=0.0  samptime=-1  NumDelays=10  DelayOrder=Oldest  includeCurrent=off
  angle : Outport
  wires:
  Tapped Delay/1 -> Sum of Elements/1
  In1/1 -> Tapped Delay/1
  Divide/1 -> angle/1
  Sum of Elements/1 -> Divide/1
  Constant/1 -> Divide/2
